simulink model "sumAttchPtsFnM_th"  (R2018b)
settings: Solver=VariableStepAuto  StartTime=0.0  StopTime=0  RelTol=1e-3
values from neighbouring files (symbols this model uses):
  euler_test = [0;0;0]    [sumAttchPtsFnM_ts.m]
  f_test = [zeros(2,n_t); ones(1,n_t)]    [sumAttchPtsFnM_ts.m]
libraries: sumAttchPtsFnM_ul x1
settings Model: Creator=asiddiq2  LastModifiedBy=asiddiq2

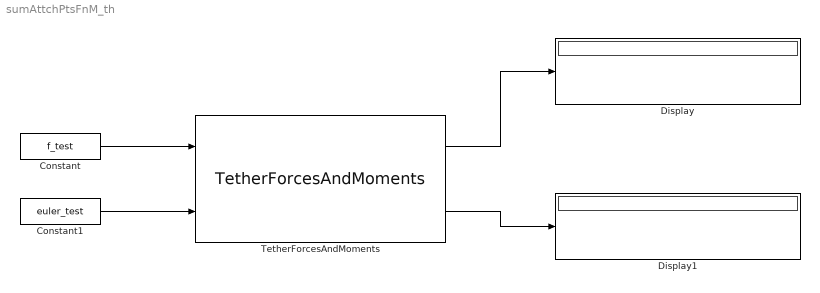
== system sumAttchPtsFnM_th ==
  Constant : Constant  Value=f_test
  Constant1 : Constant  Value=euler_test
  Display : Display
  Display1 : Display
  TetherForcesAndMoments : sumAttchPtsFnM_ul/TetherForcesAndMoments  cls_obj=some_class
  wires:
  Constant1/1 -> TetherForcesAndMoments/2
  Constant/1 -> TetherForcesAndMoments/1
  TetherForcesAndMoments/1 -> Display/1
  TetherForcesAndMoments/2 -> Display1/1
